simulink model "Peristaltic_pumps"  (R2021a)
settings: Solver=VariableStepAuto  StartTime=0.0  StopTime=50  RelTol=1e-3
libraries: fl_lib x20, nesl_utility x12, sh_lib x4
settings Model: Creator=Tomás  LastModifiedBy=ronal
settings SolverCC: AlgebraicLoopSolver=TrustRegion
settings OptimizationCC: LifeSpan=inf
settings DebuggingCC: SFExecutionAtInitializationDiag=none  SFMachineParentedDataDiag=warning  ArithmeticOperatorsInVariantConditions=warning
settings SFSimCC: CustomCodeUndefinedFunction=UseInterfaceOnly
settings CodeAppCC: StateflowObjectComments=on

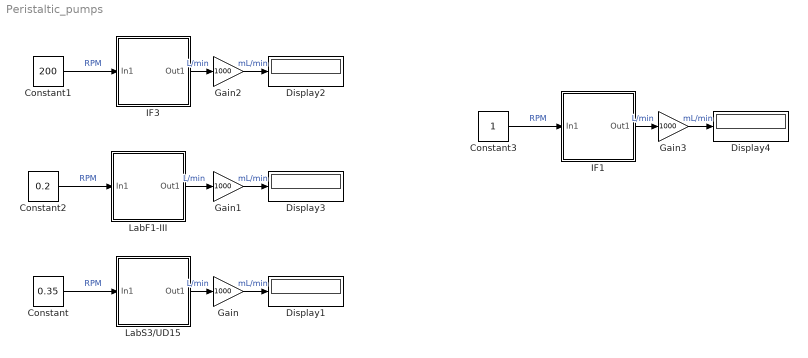
== system Peristaltic_pumps ==
  Constant : Constant  Value=0.35
  Constant1 : Constant  Value=200
  Constant2 : Constant  Value=0.2
  Constant3 : Constant
  Display{1..4} (4 alike) : Display
  Gain{,1..3} (4 alike) : Gain  Gain=1000
  IF1 : Subsystem  mask{D=0.0124, MaxRPM=350, MaxLPM=4.34, OutP=0.1, FluidDens=997, KinemVisc=0.893e-6, BulkMod=2.2e+9}
      mask prompts: D "Displacement [L/rev]"; MaxRPM "RPM Máximas [RPM]"; MaxLPM "Caudal Máximo [L/min]"; OutP "Presión de Salida [MPa]"; FluidDens "Densidad del Fluido [kg/m^3]"; KinemVisc "Viscosidad Cinemática del Fluido [m^2/s]"; BulkMod "Modulo de Compresibilidad del Fluido [Pa]"
      mask help:
      | Simulación de una Bomba Peristáltica utilizando el paquete Simscape (puede entrar en el subsistema para ver en base a que bloques se construyó).
      |
      | El principal parámetro es el Displacement, que representa cuánto aumenta el flujo de la bomba medido en Litros por Minuto [L/min] según el aumento unitario de Revoluciones por Minuto [RPM].
      |
      | El input de este bloque es una fuente de revoluciones en unidades de RPM, el cual entrega un output de caudal en L/min.
      |
      | El valor del Displacement no puede superar su valor máximo según los parámetros entregados de la bomba.
      mask Display:
      | image('bomba3.png'); % Use "Edit Image" on toolstrip to change.
      | % Bloque creado por Tomás Pröschle Donoso - DCP 2020-2
  IF3 : Subsystem  mask{D=0.0124, MaxRPM=350, MaxLPM=4.34, OutP=0.1, FluidDens=997, KinemVisc=0.893e-6, BulkMod=2.2e+9}
      mask prompts: D "Displacement [L/rev]"; MaxRPM "RPM Máximas [RPM]"; MaxLPM "Caudal Máximo [L/min]"; OutP "Presión de Salida [MPa]"; FluidDens "Densidad del Fluido [kg/m^3]"; KinemVisc "Viscosidad Cinemática del Fluido [m^2/s]"; BulkMod "Modulo de Compresibilidad del Fluido [Pa]"
      mask help:
      | Simulación de una Bomba Peristáltica utilizando el paquete Simscape (puede entrar en el subsistema para ver en base a que bloques se construyó).
      |
      | El principal parámetro es el Displacement, que representa cuánto aumenta el flujo de la bomba medido en Litros por Minuto [L/min] según el aumento unitario de Revoluciones por Minuto [RPM].
      |
      | El input de este bloque es una fuente de revoluciones en unidades de RPM, el cual entrega un output de caudal en L/min.
      |
      | El valor del Displacement no puede superar su valor máximo según los parámetros entregados de la bomba.
      mask Display:
      | image('bomba3.png'); % Use "Edit Image" on toolstrip to change.
      | % Bloque creado por Tomás Pröschle Donoso - DCP 2020-2
  LabF1-III : Subsystem  mask{D=0.00516667, MaxRPM=150, MaxLPM=0.775, OutP=0.1, FluidDens=997, KinemVisc=0.893e-6, BulkMod=2.2e+9}
      mask prompts: D "Displacement [L/rev]"; MaxRPM "RPM Máximas [RPM]"; MaxLPM "Caudal Máximo [L/min]"; OutP "Presión de Salida [MPa]"; FluidDens "Densidad del Fluido [kg/m^3]"; KinemVisc "Viscosidad Cinemática del Fluido [m^2/s]"; BulkMod "Modulo de Compresibilidad del Fluido [Pa]"
      mask help:
      | Simulación de una Bomba Peristáltica utilizando el paquete Simscape (puede entrar en el subsistema para ver en base a que bloques se construyó).
      |
      | El principal parámetro es el Displacement, que representa cuánto aumenta el flujo de la bomba medido en Litros por Minuto [L/min] según el aumento unitario de Revoluciones por Minuto [RPM].
      |
      | El input de este bloque es una fuente de revoluciones en unidades de RPM, el cual entrega un output de caudal en L/min.
      |
      | El valor del Displacement no puede superar su valor máximo según los parámetros entregados de la bomba.
      mask Display:
      | image('bomba2.png'); % Use "Edit Image" on toolstrip to change.
      | % Bloque creado por Tomás Pröschle Donoso - DCP 2020-2
  LabS3/UD15 : Subsystem  mask{D=0.0031, MaxRPM=300, MaxLPM=0.93, OutP=0.1, FluidDens=997, KinemVisc=0.893e-6, BulkMod=2.2e+9}
      mask prompts: D "Displacement [L/rev]"; MaxRPM "RPM Máximas [RPM]"; MaxLPM "Caudal Máximo [L/min]"; OutP "Presión de Salida [MPa]"; FluidDens "Densidad del Fluido [kg/m^3]"; KinemVisc "Viscosidad Cinemática del Fluido [m^2/s]"; BulkMod "Modulo de Compresibilidad del Fluido [Pa]"
      mask help:
      | Simulación de una Bomba Peristáltica utilizando el paquete Simscape (puede entrar en el subsistema para ver en base a que bloques se construyó).
      |
      | El principal parámetro es el Displacement, que representa cuánto aumenta el flujo de la bomba medido en Litros por Minuto [L/min] según el aumento unitario de Revoluciones por Minuto [RPM].
      |
      | El input de este bloque es una fuente de revoluciones en unidades de RPM, el cual entrega un output de caudal en L/min.
      |
      | El valor del Displacement no puede superar su valor máximo según los parámetros entregados de la bomba.
      mask Display:
      | image('bomba1.png'); % Use "Edit Image" on toolstrip to change.
      | % Bloque creado por Tomás Pröschle Donoso - DCP 2020-2
  wires:
  LabS3/UD15/1(Out1) -> Gain/1  "L/min"
  Constant/1 -> LabS3/UD15/1(In1)  "RPM"
  Constant1/1 -> IF3/1(In1)  "RPM"
  Constant2/1 -> LabF1-III/1(In1)  "RPM"
  Gain/1 -> Display1/1  "mL/min"
  Gain1/1 -> Display3/1  "mL/min"
  LabF1-III/1(Out1) -> Gain1/1  "L/min"
  Gain2/1 -> Display2/1  "mL/min"
  IF3/1(Out1) -> Gain2/1  "L/min"
  Gain3/1 -> Display4/1  "mL/min"
  IF1/1(Out1) -> Gain3/1  "L/min"
  Constant3/1 -> IF1/1(In1)  "RPM"

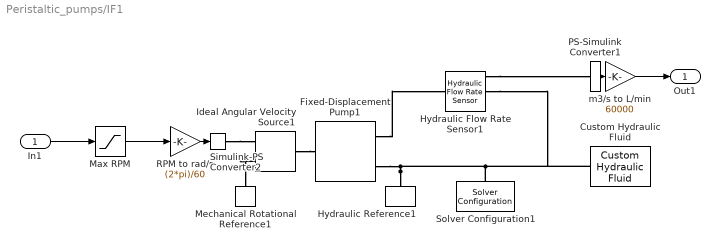
== system Peristaltic_pumps/IF1 ==
  In1 : Inport
  Custom Hydraulic Fluid : fl_lib/Hydraulic/Hydraulic Utilities/Custom Hydraulic Fluid  density=FluidDens kg/m^3  viscosity_kin=KinemVisc m^2/s  bulk=BulkMod Pa  alpha=0  range_error=2
      settings: SourceProductBaseCode=SS  InternalSimscapePortConfiguration="{\"Bottom\":[],\"Left\":[],\"Right\":[{\"id\":\"G\",\"label\":\"\",\"type\":\"foundation.hydraulic.hydraulic\"}],\"Top\":[]}"
  Fixed-Displacement Pump1 : sh_lib/Pumps and Motors/Fixed-Displacement Pump  D=D l/rev  loss_spec=1  w_nominal=MaxRPM rpm  pr_nominal=OutP MPa  visc_nominal=KinemVisc m^2/s  dens_nominal=FluidDens kg/m^3  efficiency_vol=1  no_load_torque=0 N*m  torque_pressure_coeff=0 N*m/Pa  p_diff_eff_TLU=[100000, 1000000, 2000000] Pa  omega_eff_TLU=[25, 50, 100, 200, 300, 400] rad/s  vol_eff_TLU=[.816, .908, .954, .977, .981, .984; .325, .663, .831, .916, .925, .946; .137, .568, .78, .892, .893, .91]  mech_eff_TLU=[.996, .996, .996, .996, .996, .996; .988, .989, .989, .989, .989, .99; .981, .981, .982, .982, .983, .984]  p_diff_loss_TLU=[100000, 1000000, 2000000] Pa  omega_loss_TLU=[25, 50, 100, 200, 300, 400] rad/s  vol_loss_TLU=[.023, .023, .023, .023, .0285, .032; .0844, .0842, .0845, .084, .1125, .108; .1079, .108, .11, .108, .1605, .18] * 1e-3 m^3/s  mech_loss_TLU=[.002, .002, .002, .002, .002, .002; .0607, .0556, .0556, .0556, .0556, .0505; .1937, .1937, .1833, .1833, .1729, .1626] N*m  pressure_threshold=1e5 Pa  omega_threshold=10 rad/s  quadrant_check=0  pressure_check=0  min_valid_pressure=0 Pa  vol_eff_min=1e-3  vol_eff_max=1  mech_eff_min=1e-3  mech_eff_max=1
      settings: SourceProductBaseCode=SH  InternalSimscapePortConfiguration="{\"Bottom\":[],\"Left\":[{\"id\":\"S\",\"label\":\"S\",\"type\":\"foundation.mechanical.rotational.rotational\"}],\"Right\":[{\"id\":\"P\",\"label\":\"P\",\"type\":\"foundation.hydraulic.hydraulic\"},{\"id\":\"T\",\"label\":\"T\",\"type\":\"foundation.hydraulic.hydraulic\"}],\"Top\":[]}"
  Hydraulic Flow Rate Sensor1 : fl_lib/Hydraulic/Hydraulic Sensors/Hydraulic Flow Rate Sensor
  Hydraulic Reference1 : fl_lib/Hydraulic/Hydraulic Elements/Hydraulic Reference
  Ideal Angular Velocity Source1 : fl_lib/Mechanical/Mechanical Sources/Ideal Angular Velocity Source
  Max RPM : Saturate  UpperLimit=600  LowerLimit=0
  Mechanical Rotational Reference1 : fl_lib/Mechanical/Rotational Elements/Mechanical Rotational Reference
  PS-Simulink Converter1 : nesl_utility/PS-Simulink Converter  PhysicalDomain=network_engine_domain  SubClassName=ps_output  LeftPortType=input  RightPortType=output  PseudoPeriodic=off  Frequencies=[]  Unit=inherit  AffineConversion=off
      settings: SourceProductBaseCode=PW,SS
  RPM to rad/s : Gain  Gain=(2*pi)/60
  Simulink-PS Converter2 : nesl_utility/Simulink-PS Converter  PhysicalDomain=network_engine_domain  SubClassName=ps_input  LeftPortType=input  RightPortType=output  PseudoPeriodic=off  Frequencies=[]  NoiseDistribution=none  NoiseParameters=[]  Unit=1  AffineConversion=off  FilteringAndDerivatives=provide  SimscapeFilterOrder=1  InputFilterTimeConstant=0.001  UdotUserProvided=0
      settings: SourceProductBaseCode=PW,SS
  Solver Configuration1 : nesl_utility/Solver Configuration  PhysicalDomain=network_engine_domain  SubClassName=solver  LeftPortType=input  RightPortType=generic  Tones=[]  Harmonics=[]  SimulateNoise=off  Profile=off  UseLocalSampling=off  EnableSwitchedLinearOptims=on  FrequencyDomain=off  UseCCode=off  RelTol=0.001  AbsTol=1e-06  MinStep=1e-09  ToWorkspace=off  RevertToSquareIcSolve=off  NumHomotopyIterations=100  PhasorMode=off  PhasorModeNumHarmonics=1  DoDC=off  ResidualTolerance=1e-09  UseLocalSolver=off  LocalSolverChoice=NE_BACKWARD_EULER_ADVANCER  LocalSolverSampleTime=0.001  DoFixedCost=off  MaxNonlinIter=3  MaxModeIter=2  ComputeImpulses=off  ImpulseIterations=2  LinearAlgebra=auto  EquationFormulation=NE_TIME_EF  DelaysMemoryBudget=1024  AutomaticFiltering=on  FilteringTimeConstant=0.001  PartitionStorageMethod=AS_NEEDED  PartitionMemoryBudget=1024  PartitionMethod=ROBUST
      settings: SourceProductBaseCode=PW,SS
  m3/s to L/min : Gain  Gain=60000
  Out1 : Outport
  wires:
  RPM to rad/s/1 -> Simulink-PS Converter2/1
  PS-Simulink Converter1/1 -> m3/s to L/min/1
  In1/1 -> Max RPM/1
  m3/s to L/min/1 -> Out1/1
  Max RPM/1 -> RPM to rad/s/1
  connections:
  Hydraulic Reference1/LConn1 -- Custom Hydraulic Fluid/RConn1 -- Hydraulic Flow Rate Sensor1/RConn2 -- Solver Configuration1/RConn1 -- Fixed-Displacement Pump1/RConn2
  Simulink-PS Converter2/RConn1 -- Ideal Angular Velocity Source1/RConn1
  Ideal Angular Velocity Source1/RConn2 -- Mechanical Rotational Reference1/LConn1
  Hydraulic Flow Rate Sensor1/RConn1 -- PS-Simulink Converter1/LConn1
  Fixed-Displacement Pump1/RConn1 -- Hydraulic Flow Rate Sensor1/LConn1
  Ideal Angular Velocity Source1/LConn1 -- Fixed-Displacement Pump1/LConn1

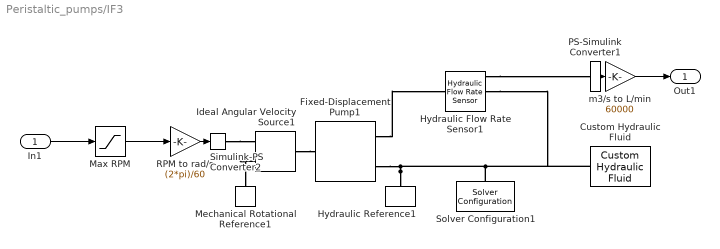
== system Peristaltic_pumps/IF3 ==
  In1 : Inport
  Custom Hydraulic Fluid : fl_lib/Hydraulic/Hydraulic Utilities/Custom Hydraulic Fluid  density=FluidDens kg/m^3  viscosity_kin=KinemVisc m^2/s  bulk=BulkMod Pa  alpha=0  range_error=2
      settings: SourceProductBaseCode=SS  InternalSimscapePortConfiguration="{\"Bottom\":[],\"Left\":[],\"Right\":[{\"id\":\"G\",\"label\":\"\",\"type\":\"foundation.hydraulic.hydraulic\"}],\"Top\":[]}"
  Fixed-Displacement Pump1 : sh_lib/Pumps and Motors/Fixed-Displacement Pump  D=D l/rev  loss_spec=1  w_nominal=MaxRPM rpm  pr_nominal=OutP MPa  visc_nominal=KinemVisc m^2/s  dens_nominal=FluidDens kg/m^3  efficiency_vol=1  no_load_torque=0 N*m  torque_pressure_coeff=0 N*m/Pa  p_diff_eff_TLU=[100000, 1000000, 2000000] Pa  omega_eff_TLU=[25, 50, 100, 200, 300, 400] rad/s  vol_eff_TLU=[.816, .908, .954, .977, .981, .984; .325, .663, .831, .916, .925, .946; .137, .568, .78, .892, .893, .91]  mech_eff_TLU=[.996, .996, .996, .996, .996, .996; .988, .989, .989, .989, .989, .99; .981, .981, .982, .982, .983, .984]  p_diff_loss_TLU=[100000, 1000000, 2000000] Pa  omega_loss_TLU=[25, 50, 100, 200, 300, 400] rad/s  vol_loss_TLU=[.023, .023, .023, .023, .0285, .032; .0844, .0842, .0845, .084, .1125, .108; .1079, .108, .11, .108, .1605, .18] * 1e-3 m^3/s  mech_loss_TLU=[.002, .002, .002, .002, .002, .002; .0607, .0556, .0556, .0556, .0556, .0505; .1937, .1937, .1833, .1833, .1729, .1626] N*m  pressure_threshold=1e5 Pa  omega_threshold=10 rad/s  quadrant_check=0  pressure_check=0  min_valid_pressure=0 Pa  vol_eff_min=1e-3  vol_eff_max=1  mech_eff_min=1e-3  mech_eff_max=1
      settings: SourceProductBaseCode=SH  InternalSimscapePortConfiguration="{\"Bottom\":[],\"Left\":[{\"id\":\"S\",\"label\":\"S\",\"type\":\"foundation.mechanical.rotational.rotational\"}],\"Right\":[{\"id\":\"P\",\"label\":\"P\",\"type\":\"foundation.hydraulic.hydraulic\"},{\"id\":\"T\",\"label\":\"T\",\"type\":\"foundation.hydraulic.hydraulic\"}],\"Top\":[]}"
  Hydraulic Flow Rate Sensor1 : fl_lib/Hydraulic/Hydraulic Sensors/Hydraulic Flow Rate Sensor
  Hydraulic Reference1 : fl_lib/Hydraulic/Hydraulic Elements/Hydraulic Reference
  Ideal Angular Velocity Source1 : fl_lib/Mechanical/Mechanical Sources/Ideal Angular Velocity Source
  Max RPM : Saturate  UpperLimit=600  LowerLimit=0
  Mechanical Rotational Reference1 : fl_lib/Mechanical/Rotational Elements/Mechanical Rotational Reference
  PS-Simulink Converter1 : nesl_utility/PS-Simulink Converter  PhysicalDomain=network_engine_domain  SubClassName=ps_output  LeftPortType=input  RightPortType=output  PseudoPeriodic=off  Frequencies=[]  Unit=inherit  AffineConversion=off
      settings: SourceProductBaseCode=PW,SS
  RPM to rad/s : Gain  Gain=(2*pi)/60
  Simulink-PS Converter2 : nesl_utility/Simulink-PS Converter  PhysicalDomain=network_engine_domain  SubClassName=ps_input  LeftPortType=input  RightPortType=output  PseudoPeriodic=off  Frequencies=[]  NoiseDistribution=none  NoiseParameters=[]  Unit=1  AffineConversion=off  FilteringAndDerivatives=provide  SimscapeFilterOrder=1  InputFilterTimeConstant=0.001  UdotUserProvided=0
      settings: SourceProductBaseCode=PW,SS
  Solver Configuration1 : nesl_utility/Solver Configuration  PhysicalDomain=network_engine_domain  SubClassName=solver  LeftPortType=input  RightPortType=generic  Tones=[]  Harmonics=[]  SimulateNoise=off  Profile=off  UseLocalSampling=off  EnableSwitchedLinearOptims=on  FrequencyDomain=off  UseCCode=off  RelTol=0.001  AbsTol=1e-06  MinStep=1e-09  ToWorkspace=off  RevertToSquareIcSolve=off  NumHomotopyIterations=100  PhasorMode=off  PhasorModeNumHarmonics=1  DoDC=off  ResidualTolerance=1e-09  UseLocalSolver=off  LocalSolverChoice=NE_BACKWARD_EULER_ADVANCER  LocalSolverSampleTime=0.001  DoFixedCost=off  MaxNonlinIter=3  MaxModeIter=2  ComputeImpulses=off  ImpulseIterations=2  LinearAlgebra=auto  EquationFormulation=NE_TIME_EF  DelaysMemoryBudget=1024  AutomaticFiltering=on  FilteringTimeConstant=0.001  PartitionStorageMethod=AS_NEEDED  PartitionMemoryBudget=1024  PartitionMethod=ROBUST
      settings: SourceProductBaseCode=PW,SS
  m3/s to L/min : Gain  Gain=60000
  Out1 : Outport
  wires:
  RPM to rad/s/1 -> Simulink-PS Converter2/1
  PS-Simulink Converter1/1 -> m3/s to L/min/1
  In1/1 -> Max RPM/1
  m3/s to L/min/1 -> Out1/1
  Max RPM/1 -> RPM to rad/s/1
  connections:
  Hydraulic Reference1/LConn1 -- Custom Hydraulic Fluid/RConn1 -- Hydraulic Flow Rate Sensor1/RConn2 -- Solver Configuration1/RConn1 -- Fixed-Displacement Pump1/RConn2
  Simulink-PS Converter2/RConn1 -- Ideal Angular Velocity Source1/RConn1
  Ideal Angular Velocity Source1/RConn2 -- Mechanical Rotational Reference1/LConn1
  Hydraulic Flow Rate Sensor1/RConn1 -- PS-Simulink Converter1/LConn1
  Fixed-Displacement Pump1/RConn1 -- Hydraulic Flow Rate Sensor1/LConn1
  Ideal Angular Velocity Source1/LConn1 -- Fixed-Displacement Pump1/LConn1

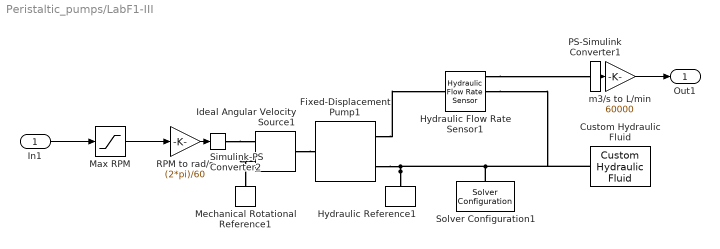
== system Peristaltic_pumps/LabF1-III ==
  In1 : Inport
  Custom Hydraulic Fluid : fl_lib/Hydraulic/Hydraulic Utilities/Custom Hydraulic Fluid  density=FluidDens kg/m^3  viscosity_kin=KinemVisc m^2/s  bulk=BulkMod Pa  alpha=0  range_error=2
      settings: SourceProductBaseCode=SS  InternalSimscapePortConfiguration="{\"Bottom\":[],\"Left\":[],\"Right\":[{\"id\":\"G\",\"label\":\"\",\"type\":\"foundation.hydraulic.hydraulic\"}],\"Top\":[]}"
  Fixed-Displacement Pump1 : sh_lib/Pumps and Motors/Fixed-Displacement Pump  D=D l/rev  loss_spec=1  w_nominal=MaxRPM rpm  pr_nominal=OutP MPa  visc_nominal=KinemVisc m^2/s  dens_nominal=FluidDens kg/m^3  efficiency_vol=1  no_load_torque=0 N*m  torque_pressure_coeff=0 N*m/Pa  p_diff_eff_TLU=[100000, 1000000, 2000000] Pa  omega_eff_TLU=[25, 50, 100, 200, 300, 400] rad/s  vol_eff_TLU=[.816, .908, .954, .977, .981, .984; .325, .663, .831, .916, .925, .946; .137, .568, .78, .892, .893, .91]  mech_eff_TLU=[.996, .996, .996, .996, .996, .996; .988, .989, .989, .989, .989, .99; .981, .981, .982, .982, .983, .984]  p_diff_loss_TLU=[100000, 1000000, 2000000] Pa  omega_loss_TLU=[25, 50, 100, 200, 300, 400] rad/s  vol_loss_TLU=[.023, .023, .023, .023, .0285, .032; .0844, .0842, .0845, .084, .1125, .108; .1079, .108, .11, .108, .1605, .18] * 1e-3 m^3/s  mech_loss_TLU=[.002, .002, .002, .002, .002, .002; .0607, .0556, .0556, .0556, .0556, .0505; .1937, .1937, .1833, .1833, .1729, .1626] N*m  pressure_threshold=1e5 Pa  omega_threshold=10 rad/s  quadrant_check=0  pressure_check=0  min_valid_pressure=0 Pa  vol_eff_min=1e-3  vol_eff_max=1  mech_eff_min=1e-3  mech_eff_max=1
      settings: SourceProductBaseCode=SH  InternalSimscapePortConfiguration="{\"Bottom\":[],\"Left\":[{\"id\":\"S\",\"label\":\"S\",\"type\":\"foundation.mechanical.rotational.rotational\"}],\"Right\":[{\"id\":\"P\",\"label\":\"P\",\"type\":\"foundation.hydraulic.hydraulic\"},{\"id\":\"T\",\"label\":\"T\",\"type\":\"foundation.hydraulic.hydraulic\"}],\"Top\":[]}"
  Hydraulic Flow Rate Sensor1 : fl_lib/Hydraulic/Hydraulic Sensors/Hydraulic Flow Rate Sensor
  Hydraulic Reference1 : fl_lib/Hydraulic/Hydraulic Elements/Hydraulic Reference
  Ideal Angular Velocity Source1 : fl_lib/Mechanical/Mechanical Sources/Ideal Angular Velocity Source
  Max RPM : Saturate  UpperLimit=600  LowerLimit=0
  Mechanical Rotational Reference1 : fl_lib/Mechanical/Rotational Elements/Mechanical Rotational Reference
  PS-Simulink Converter1 : nesl_utility/PS-Simulink Converter  PhysicalDomain=network_engine_domain  SubClassName=ps_output  LeftPortType=input  RightPortType=output  PseudoPeriodic=off  Frequencies=[]  Unit=inherit  AffineConversion=off
      settings: SourceProductBaseCode=PW,SS
  RPM to rad/s : Gain  Gain=(2*pi)/60
  Simulink-PS Converter2 : nesl_utility/Simulink-PS Converter  PhysicalDomain=network_engine_domain  SubClassName=ps_input  LeftPortType=input  RightPortType=output  PseudoPeriodic=off  Frequencies=[]  NoiseDistribution=none  NoiseParameters=[]  Unit=1  AffineConversion=off  FilteringAndDerivatives=provide  SimscapeFilterOrder=1  InputFilterTimeConstant=0.001  UdotUserProvided=0
      settings: SourceProductBaseCode=PW,SS
  Solver Configuration1 : nesl_utility/Solver Configuration  PhysicalDomain=network_engine_domain  SubClassName=solver  LeftPortType=input  RightPortType=generic  Tones=[]  Harmonics=[]  SimulateNoise=off  Profile=off  UseLocalSampling=off  EnableSwitchedLinearOptims=on  FrequencyDomain=off  UseCCode=off  RelTol=0.001  AbsTol=1e-06  MinStep=1e-09  ToWorkspace=off  RevertToSquareIcSolve=off  NumHomotopyIterations=100  PhasorMode=off  PhasorModeNumHarmonics=1  DoDC=off  ResidualTolerance=1e-09  UseLocalSolver=off  LocalSolverChoice=NE_BACKWARD_EULER_ADVANCER  LocalSolverSampleTime=0.001  DoFixedCost=off  MaxNonlinIter=3  MaxModeIter=2  ComputeImpulses=off  ImpulseIterations=2  LinearAlgebra=auto  EquationFormulation=NE_TIME_EF  DelaysMemoryBudget=1024  AutomaticFiltering=on  FilteringTimeConstant=0.001  PartitionStorageMethod=AS_NEEDED  PartitionMemoryBudget=1024  PartitionMethod=ROBUST
      settings: SourceProductBaseCode=PW,SS
  m3/s to L/min : Gain  Gain=60000
  Out1 : Outport
  wires:
  RPM to rad/s/1 -> Simulink-PS Converter2/1
  PS-Simulink Converter1/1 -> m3/s to L/min/1
  In1/1 -> Max RPM/1
  m3/s to L/min/1 -> Out1/1
  Max RPM/1 -> RPM to rad/s/1
  connections:
  Hydraulic Reference1/LConn1 -- Custom Hydraulic Fluid/RConn1 -- Hydraulic Flow Rate Sensor1/RConn2 -- Solver Configuration1/RConn1 -- Fixed-Displacement Pump1/RConn2
  Simulink-PS Converter2/RConn1 -- Ideal Angular Velocity Source1/RConn1
  Ideal Angular Velocity Source1/RConn2 -- Mechanical Rotational Reference1/LConn1
  Hydraulic Flow Rate Sensor1/RConn1 -- PS-Simulink Converter1/LConn1
  Fixed-Displacement Pump1/RConn1 -- Hydraulic Flow Rate Sensor1/LConn1
  Ideal Angular Velocity Source1/LConn1 -- Fixed-Displacement Pump1/LConn1

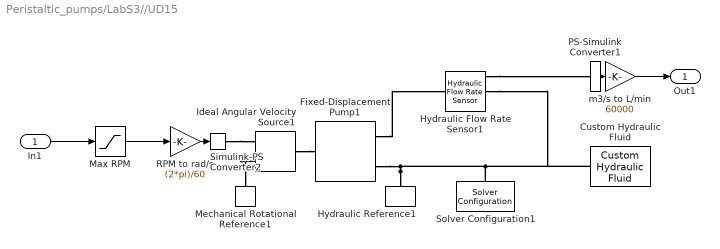
== system Peristaltic_pumps/LabS3//UD15 ==
  In1 : Inport
  Custom Hydraulic Fluid : fl_lib/Hydraulic/Hydraulic Utilities/Custom Hydraulic Fluid  density=FluidDens kg/m^3  viscosity_kin=KinemVisc m^2/s  bulk=BulkMod Pa  alpha=0  range_error=2
      settings: SourceProductBaseCode=SS  InternalSimscapePortConfiguration="{\"Bottom\":[],\"Left\":[],\"Right\":[{\"id\":\"G\",\"label\":\"\",\"type\":\"foundation.hydraulic.hydraulic\"}],\"Top\":[]}"
  Fixed-Displacement Pump1 : sh_lib/Pumps and Motors/Fixed-Displacement Pump  D=D l/rev  loss_spec=1  w_nominal=MaxRPM rpm  pr_nominal=OutP MPa  visc_nominal=KinemVisc m^2/s  dens_nominal=FluidDens kg/m^3  efficiency_vol=1  no_load_torque=0 N*m  torque_pressure_coeff=0 N*m/Pa  p_diff_eff_TLU=[100000, 1000000, 2000000] Pa  omega_eff_TLU=[25, 50, 100, 200, 300, 400] rad/s  vol_eff_TLU=[.816, .908, .954, .977, .981, .984; .325, .663, .831, .916, .925, .946; .137, .568, .78, .892, .893, .91]  mech_eff_TLU=[.996, .996, .996, .996, .996, .996; .988, .989, .989, .989, .989, .99; .981, .981, .982, .982, .983, .984]  p_diff_loss_TLU=[100000, 1000000, 2000000] Pa  omega_loss_TLU=[25, 50, 100, 200, 300, 400] rad/s  vol_loss_TLU=[.023, .023, .023, .023, .0285, .032; .0844, .0842, .0845, .084, .1125, .108; .1079, .108, .11, .108, .1605, .18] * 1e-3 m^3/s  mech_loss_TLU=[.002, .002, .002, .002, .002, .002; .0607, .0556, .0556, .0556, .0556, .0505; .1937, .1937, .1833, .1833, .1729, .1626] N*m  pressure_threshold=1e5 Pa  omega_threshold=10 rad/s  quadrant_check=0  pressure_check=0  min_valid_pressure=0 Pa  vol_eff_min=1e-3  vol_eff_max=1  mech_eff_min=1e-3  mech_eff_max=1
      settings: SourceProductBaseCode=SH  InternalSimscapePortConfiguration="{\"Bottom\":[],\"Left\":[{\"id\":\"S\",\"label\":\"S\",\"type\":\"foundation.mechanical.rotational.rotational\"}],\"Right\":[{\"id\":\"P\",\"label\":\"P\",\"type\":\"foundation.hydraulic.hydraulic\"},{\"id\":\"T\",\"label\":\"T\",\"type\":\"foundation.hydraulic.hydraulic\"}],\"Top\":[]}"
  Hydraulic Flow Rate Sensor1 : fl_lib/Hydraulic/Hydraulic Sensors/Hydraulic Flow Rate Sensor
  Hydraulic Reference1 : fl_lib/Hydraulic/Hydraulic Elements/Hydraulic Reference
  Ideal Angular Velocity Source1 : fl_lib/Mechanical/Mechanical Sources/Ideal Angular Velocity Source
  Max RPM : Saturate  UpperLimit=600  LowerLimit=0
  Mechanical Rotational Reference1 : fl_lib/Mechanical/Rotational Elements/Mechanical Rotational Reference
  PS-Simulink Converter1 : nesl_utility/PS-Simulink Converter  PhysicalDomain=network_engine_domain  SubClassName=ps_output  LeftPortType=input  RightPortType=output  PseudoPeriodic=off  Frequencies=[]  Unit=inherit  AffineConversion=off
      settings: SourceProductBaseCode=PW,SS
  RPM to rad/s : Gain  Gain=(2*pi)/60
  Simulink-PS Converter2 : nesl_utility/Simulink-PS Converter  PhysicalDomain=network_engine_domain  SubClassName=ps_input  LeftPortType=input  RightPortType=output  PseudoPeriodic=off  Frequencies=[]  NoiseDistribution=none  NoiseParameters=[]  Unit=1  AffineConversion=off  FilteringAndDerivatives=provide  SimscapeFilterOrder=1  InputFilterTimeConstant=0.001  UdotUserProvided=0
      settings: SourceProductBaseCode=PW,SS
  Solver Configuration1 : nesl_utility/Solver Configuration  PhysicalDomain=network_engine_domain  SubClassName=solver  LeftPortType=input  RightPortType=generic  Tones=[]  Harmonics=[]  SimulateNoise=off  Profile=off  UseLocalSampling=off  EnableSwitchedLinearOptims=on  FrequencyDomain=off  UseCCode=off  RelTol=0.001  AbsTol=1e-06  MinStep=1e-09  ToWorkspace=off  RevertToSquareIcSolve=off  NumHomotopyIterations=100  PhasorMode=off  PhasorModeNumHarmonics=1  DoDC=off  ResidualTolerance=1e-09  UseLocalSolver=off  LocalSolverChoice=NE_BACKWARD_EULER_ADVANCER  LocalSolverSampleTime=0.001  DoFixedCost=off  MaxNonlinIter=3  MaxModeIter=2  ComputeImpulses=off  ImpulseIterations=2  LinearAlgebra=auto  EquationFormulation=NE_TIME_EF  DelaysMemoryBudget=1024  AutomaticFiltering=on  FilteringTimeConstant=0.001  PartitionStorageMethod=AS_NEEDED  PartitionMemoryBudget=1024  PartitionMethod=ROBUST
      settings: SourceProductBaseCode=PW,SS
  m3/s to L/min : Gain  Gain=60000
  Out1 : Outport
  wires:
  RPM to rad/s/1 -> Simulink-PS Converter2/1
  PS-Simulink Converter1/1 -> m3/s to L/min/1
  In1/1 -> Max RPM/1
  m3/s to L/min/1 -> Out1/1
  Max RPM/1 -> RPM to rad/s/1
  connections:
  Hydraulic Reference1/LConn1 -- Custom Hydraulic Fluid/RConn1 -- Hydraulic Flow Rate Sensor1/RConn2 -- Solver Configuration1/RConn1 -- Fixed-Displacement Pump1/RConn2
  Simulink-PS Converter2/RConn1 -- Ideal Angular Velocity Source1/RConn1
  Ideal Angular Velocity Source1/RConn2 -- Mechanical Rotational Reference1/LConn1
  Hydraulic Flow Rate Sensor1/RConn1 -- PS-Simulink Converter1/LConn1
  Fixed-Displacement Pump1/RConn1 -- Hydraulic Flow Rate Sensor1/LConn1
  Ideal Angular Velocity Source1/LConn1 -- Fixed-Displacement Pump1/LConn1
